simulink model "ASM_Traffic_V2X_Complete_Model_2"  (R2019a)
settings: Solver=ode1  StartTime=SIM.tstart.v  StopTime=Inf  FixedStep=SIM.StepSize.v  RelTol=1e-3
PostLoadFcn:
  | if any(exist('dsrtsu_mdlpostloadfcn', 'file') ~= 0), dsrtsu_mdlpostloadfcn('Execute', bdroot); end
  | try, asm_mdl_postloadfcn(bdroot, 'UpdateModel', 2200); catch, disp(lasterr); end,
undefined symbols (not defined in the file): _SensorPnts_1, _SensorPnts_13, _SensorPnts_17, _SensorPnts_21, _SensorPnts_25, _SensorPnts_29, _SensorPnts_33, _SensorPnts_37, _SensorPnts_41, _SensorPnts_45, _SensorPnts_49, _SensorPnts_5, _SensorPnts_53, _SensorPnts_57, _SensorPnts_9, _to_, CPT, G5A, ITS, MDL, rad, s_to_rpm, SIM
libraries: simulink x169, ASM_VehicleDynamics_lib x126, ASM_Traffic_lib x83, ASM_Utils_lib x49, mdbs x45, ASM_Environment_lib x17, dspindex x12, dsaV2xLibraryAux x10, dsmpblib x6, dsaV2xAsn1Library x4, dsaV2xLibrary x4, ASM_BrakeHydraulics_lib x4
(part 22 of 36)

== system ASM_Traffic_V2X_Complete_Model_2/MDLUserInterface/Environment/MDL_PAR/Fellow_VehicleLights/Fellow13_VehicleLights ==
  Bus Creator1 : BusCreator  Inputs=3
  SW_BrakeLight[0Off|1On] : Constant  Value=0
  SW_ManualControl_Lights[1Scheduler|2Manual] : Constant
  SW_TurnLights[0Off|1Left|2Right|3Both] : Constant  Value=0
  Out1 : Outport
  wires:
  SW_ManualControl_Lights[1Scheduler|2Manual]/1 -> Bus Creator1/1  "SW_ManualControl_Lights[1Scheduler|2Manual]"
  SW_TurnLights[0Off|1Left|2Right|3Both]/1 -> Bus Creator1/3  "SW_TurnLights[0Off|1Left|2Right|3Both]"
  SW_BrakeLight[0Off|1On]/1 -> Bus Creator1/2  "SW_BrakeLight[0Off|1On]"
  Bus Creator1/1 -> Out1/1

== system ASM_Traffic_V2X_Complete_Model_2/MDLUserInterface/Environment/MDL_PAR/Fellow_VehicleLights/Fellow14_VehicleLights ==
  Bus Creator1 : BusCreator  Inputs=3
  SW_BrakeLight[0Off|1On] : Constant  Value=0
  SW_ManualControl_Lights[1Scheduler|2Manual] : Constant
  SW_TurnLights[0Off|1Left|2Right|3Both] : Constant  Value=0
  Out1 : Outport
  wires:
  Bus Creator1/1 -> Out1/1
  SW_BrakeLight[0Off|1On]/1 -> Bus Creator1/2  "SW_BrakeLight[0Off|1On]"
  SW_TurnLights[0Off|1Left|2Right|3Both]/1 -> Bus Creator1/3  "SW_TurnLights[0Off|1Left|2Right|3Both]"
  SW_ManualControl_Lights[1Scheduler|2Manual]/1 -> Bus Creator1/1  "SW_ManualControl_Lights[1Scheduler|2Manual]"

== system ASM_Traffic_V2X_Complete_Model_2/MDLUserInterface/Environment/MDL_PAR/Fellow_VehicleLights/Fellow15_VehicleLights ==
  Bus Creator1 : BusCreator  Inputs=3
  SW_BrakeLight[0Off|1On] : Constant  Value=0
  SW_ManualControl_Lights[1Scheduler|2Manual] : Constant
  SW_TurnLights[0Off|1Left|2Right|3Both] : Constant  Value=0
  Out1 : Outport
  wires:
  SW_ManualControl_Lights[1Scheduler|2Manual]/1 -> Bus Creator1/1  "SW_ManualControl_Lights[1Scheduler|2Manual]"
  SW_TurnLights[0Off|1Left|2Right|3Both]/1 -> Bus Creator1/3  "SW_TurnLights[0Off|1Left|2Right|3Both]"
  SW_BrakeLight[0Off|1On]/1 -> Bus Creator1/2  "SW_BrakeLight[0Off|1On]"
  Bus Creator1/1 -> Out1/1

== system ASM_Traffic_V2X_Complete_Model_2/MDLUserInterface/Environment/MDL_PAR/Fellow_VehicleLights/Fellow1_VehicleLights ==
  Bus Creator1 : BusCreator  Inputs=3
  SW_BrakeLight[0Off|1On] : Constant  Value=0
  SW_ManualControl_Lights[1Scheduler|2Manual] : Constant
  SW_TurnLights[0Off|1Left|2Right|3Both] : Constant  Value=0
  Out1 : Outport
  wires:
  SW_ManualControl_Lights[1Scheduler|2Manual]/1 -> Bus Creator1/1  "SW_ManualControl_Lights[1Scheduler|2Manual]"
  SW_TurnLights[0Off|1Left|2Right|3Both]/1 -> Bus Creator1/3  "SW_TurnLights[0Off|1Left|2Right|3Both]"
  SW_BrakeLight[0Off|1On]/1 -> Bus Creator1/2  "SW_BrakeLight[0Off|1On]"
  Bus Creator1/1 -> Out1/1

== system ASM_Traffic_V2X_Complete_Model_2/MDLUserInterface/Environment/MDL_PAR/Fellow_VehicleLights/Fellow2_VehicleLights ==
  Bus Creator1 : BusCreator  Inputs=3
  SW_BrakeLight[0Off|1On] : Constant  Value=0
  SW_ManualControl_Lights[1Scheduler|2Manual] : Constant
  SW_TurnLights[0Off|1Left|2Right|3Both] : Constant  Value=0
  Out1 : Outport
  wires:
  Bus Creator1/1 -> Out1/1
  SW_BrakeLight[0Off|1On]/1 -> Bus Creator1/2  "SW_BrakeLight[0Off|1On]"
  SW_TurnLights[0Off|1Left|2Right|3Both]/1 -> Bus Creator1/3  "SW_TurnLights[0Off|1Left|2Right|3Both]"
  SW_ManualControl_Lights[1Scheduler|2Manual]/1 -> Bus Creator1/1  "SW_ManualControl_Lights[1Scheduler|2Manual]"

== system ASM_Traffic_V2X_Complete_Model_2/MDLUserInterface/Environment/MDL_PAR/Fellow_VehicleLights/Fellow3_VehicleLights ==
  Bus Creator1 : BusCreator  Inputs=3
  SW_BrakeLight[0Off|1On] : Constant  Value=0
  SW_ManualControl_Lights[1Scheduler|2Manual] : Constant
  SW_TurnLights[0Off|1Left|2Right|3Both] : Constant  Value=0
  Out1 : Outport
  wires:
  SW_ManualControl_Lights[1Scheduler|2Manual]/1 -> Bus Creator1/1  "SW_ManualControl_Lights[1Scheduler|2Manual]"
  SW_TurnLights[0Off|1Left|2Right|3Both]/1 -> Bus Creator1/3  "SW_TurnLights[0Off|1Left|2Right|3Both]"
  SW_BrakeLight[0Off|1On]/1 -> Bus Creator1/2  "SW_BrakeLight[0Off|1On]"
  Bus Creator1/1 -> Out1/1

== system ASM_Traffic_V2X_Complete_Model_2/MDLUserInterface/Environment/MDL_PAR/Fellow_VehicleLights/Fellow4_VehicleLights ==
  Bus Creator1 : BusCreator  Inputs=3
  SW_BrakeLight[0Off|1On] : Constant  Value=0
  SW_ManualControl_Lights[1Scheduler|2Manual] : Constant
  SW_TurnLights[0Off|1Left|2Right|3Both] : Constant  Value=0
  Out1 : Outport
  wires:
  Bus Creator1/1 -> Out1/1
  SW_BrakeLight[0Off|1On]/1 -> Bus Creator1/2  "SW_BrakeLight[0Off|1On]"
  SW_TurnLights[0Off|1Left|2Right|3Both]/1 -> Bus Creator1/3  "SW_TurnLights[0Off|1Left|2Right|3Both]"
  SW_ManualControl_Lights[1Scheduler|2Manual]/1 -> Bus Creator1/1  "SW_ManualControl_Lights[1Scheduler|2Manual]"

== system ASM_Traffic_V2X_Complete_Model_2/MDLUserInterface/Environment/MDL_PAR/Fellow_VehicleLights/Fellow5_VehicleLights ==
  Bus Creator1 : BusCreator  Inputs=3
  SW_BrakeLight[0Off|1On] : Constant  Value=0
  SW_ManualControl_Lights[1Scheduler|2Manual] : Constant
  SW_TurnLights[0Off|1Left|2Right|3Both] : Constant  Value=0
  Out1 : Outport
  wires:
  SW_ManualControl_Lights[1Scheduler|2Manual]/1 -> Bus Creator1/1  "SW_ManualControl_Lights[1Scheduler|2Manual]"
  SW_TurnLights[0Off|1Left|2Right|3Both]/1 -> Bus Creator1/3  "SW_TurnLights[0Off|1Left|2Right|3Both]"
  SW_BrakeLight[0Off|1On]/1 -> Bus Creator1/2  "SW_BrakeLight[0Off|1On]"
  Bus Creator1/1 -> Out1/1

== system ASM_Traffic_V2X_Complete_Model_2/MDLUserInterface/Environment/MDL_PAR/Fellow_VehicleLights/Fellow6_VehicleLights ==
  Bus Creator1 : BusCreator  Inputs=3
  SW_BrakeLight[0Off|1On] : Constant  Value=0
  SW_ManualControl_Lights[1Scheduler|2Manual] : Constant
  SW_TurnLights[0Off|1Left|2Right|3Both] : Constant  Value=0
  Out1 : Outport
  wires:
  Bus Creator1/1 -> Out1/1
  SW_BrakeLight[0Off|1On]/1 -> Bus Creator1/2  "SW_BrakeLight[0Off|1On]"
  SW_TurnLights[0Off|1Left|2Right|3Both]/1 -> Bus Creator1/3  "SW_TurnLights[0Off|1Left|2Right|3Both]"
  SW_ManualControl_Lights[1Scheduler|2Manual]/1 -> Bus Creator1/1  "SW_ManualControl_Lights[1Scheduler|2Manual]"

== system ASM_Traffic_V2X_Complete_Model_2/MDLUserInterface/Environment/MDL_PAR/Fellow_VehicleLights/Fellow7_VehicleLights ==
  Bus Creator1 : BusCreator  Inputs=3
  SW_BrakeLight[0Off|1On] : Constant  Value=0
  SW_ManualControl_Lights[1Scheduler|2Manual] : Constant
  SW_TurnLights[0Off|1Left|2Right|3Both] : Constant  Value=0
  Out1 : Outport
  wires:
  SW_ManualControl_Lights[1Scheduler|2Manual]/1 -> Bus Creator1/1  "SW_ManualControl_Lights[1Scheduler|2Manual]"
  SW_TurnLights[0Off|1Left|2Right|3Both]/1 -> Bus Creator1/3  "SW_TurnLights[0Off|1Left|2Right|3Both]"
  SW_BrakeLight[0Off|1On]/1 -> Bus Creator1/2  "SW_BrakeLight[0Off|1On]"
  Bus Creator1/1 -> Out1/1

== system ASM_Traffic_V2X_Complete_Model_2/MDLUserInterface/Environment/MDL_PAR/Fellow_VehicleLights/Fellow8_VehicleLights ==
  Bus Creator1 : BusCreator  Inputs=3
  SW_BrakeLight[0Off|1On] : Constant  Value=0
  SW_ManualControl_Lights[1Scheduler|2Manual] : Constant
  SW_TurnLights[0Off|1Left|2Right|3Both] : Constant  Value=0
  Out1 : Outport
  wires:
  Bus Creator1/1 -> Out1/1
  SW_BrakeLight[0Off|1On]/1 -> Bus Creator1/2  "SW_BrakeLight[0Off|1On]"
  SW_TurnLights[0Off|1Left|2Right|3Both]/1 -> Bus Creator1/3  "SW_TurnLights[0Off|1Left|2Right|3Both]"
  SW_ManualControl_Lights[1Scheduler|2Manual]/1 -> Bus Creator1/1  "SW_ManualControl_Lights[1Scheduler|2Manual]"

== system ASM_Traffic_V2X_Complete_Model_2/MDLUserInterface/Environment/MDL_PAR/Fellow_VehicleLights/Fellow9_VehicleLights ==
  Bus Creator1 : BusCreator  Inputs=3
  SW_BrakeLight[0Off|1On] : Constant  Value=0
  SW_ManualControl_Lights[1Scheduler|2Manual] : Constant
  SW_TurnLights[0Off|1Left|2Right|3Both] : Constant  Value=0
  Out1 : Outport
  wires:
  SW_ManualControl_Lights[1Scheduler|2Manual]/1 -> Bus Creator1/1  "SW_ManualControl_Lights[1Scheduler|2Manual]"
  SW_TurnLights[0Off|1Left|2Right|3Both]/1 -> Bus Creator1/3  "SW_TurnLights[0Off|1Left|2Right|3Both]"
  SW_BrakeLight[0Off|1On]/1 -> Bus Creator1/2  "SW_BrakeLight[0Off|1On]"
  Bus Creator1/1 -> Out1/1

== system ASM_Traffic_V2X_Complete_Model_2/MDLUserInterface/Environment/MDL_PAR/ManeuverControl/Enable_ManeuverStart ==
  Sw_StartManeuverAtSimStart[0|1] : Inport
  In : Inport  Port=2
  Data Type Conversion : DataTypeConversion
  Logical Operator : Logic  Operator=OR  AllPortsSameDT=off  OutDataTypeStr=boolean
  Product : Product  Inputs=3
  Step : Step  Time=0.005  SampleTime=0
  Step1 : Step  Time=0.02  Before=1  After=0  SampleTime=0
  Out : Outport
  wires:
  In/1 -> Logical Operator/1
  Data Type Conversion/1 -> Out/1
  Logical Operator/1 -> Data Type Conversion/1
  Step1/1 -> Product/3
  Product/1 -> Logical Operator/2
  Sw_StartManeuverAtSimStart[0|1]/1 -> Product/1
  Step/1 -> Product/2

== system ASM_Traffic_V2X_Complete_Model_2/MDLUserInterface/Environment/MDL_PAR/Objects_DataStreams/DataStream_1 ==
  Bus Creator1 : BusCreator  Inputs=4
  Ext_DataStream_1[] : Constant  Value=0
  Multiport Switch : MultiPortSwitch  DataPortOrder=Zero-based contiguous  Inputs=2  zeroidx=on
  Rounding Function : Rounding  Operator=round
  Saturation : Saturate  UpperLimit=2  LowerLimit=0
  Stim_DataStream_1[] : Constant
  Sw_DataStream_1[0Stim|1Ext] : Constant  Value=0
  DataStream_1[] : Outport
  wires:
  Sw_DataStream_1[0Stim|1Ext]/1 -> Rounding Function/1, Bus Creator1/1  "Sw_DataStream_1[0Stim|1Ext]"
  Ext_DataStream_1[]/1 -> Bus Creator1/3, Multiport Switch/3  "Ext_DataStream_1[]"
  Rounding Function/1 -> Saturation/1
  Saturation/1 -> Multiport Switch/1
  Multiport Switch/1 -> Bus Creator1/4  "DataStream_1[]"
  Stim_DataStream_1[]/1 -> Multiport Switch/2, Bus Creator1/2  "Stim_DataStream_1[]"
  Bus Creator1/1 -> DataStream_1[]/1

== system ASM_Traffic_V2X_Complete_Model_2/MDLUserInterface/Environment/MDL_PAR/Objects_DataStreams/DataStream_2 ==
  Bus Creator1 : BusCreator  Inputs=4
  Ext_DataStream_2[] : Constant  Value=0
  Multiport Switch : MultiPortSwitch  DataPortOrder=Zero-based contiguous  Inputs=2  zeroidx=on
  Rounding Function : Rounding  Operator=round
  Saturation : Saturate  UpperLimit=2  LowerLimit=0
  Stim_DataStream_2[] : Constant
  Sw_DataStream_2[0Stim|1Ext] : Constant  Value=0
  DataStream_2[] : Outport
  wires:
  Bus Creator1/1 -> DataStream_2[]/1
  Stim_DataStream_2[]/1 -> Bus Creator1/2, Multiport Switch/2  "Stim_DataStream_2[]"
  Multiport Switch/1 -> Bus Creator1/4  "DataStream_2[]"
  Saturation/1 -> Multiport Switch/1
  Rounding Function/1 -> Saturation/1
  Ext_DataStream_2[]/1 -> Multiport Switch/3, Bus Creator1/3  "Ext_DataStream_2[]"
  Sw_DataStream_2[0Stim|1Ext]/1 -> Bus Creator1/1, Rounding Function/1  "Sw_DataStream_2[0Stim|1Ext]"

== system ASM_Traffic_V2X_Complete_Model_2/MDLUserInterface/Environment/MDL_PAR/Objects_DataStreams/DataStream_3 ==
  Bus Creator1 : BusCreator  Inputs=4
  Ext_DataStream_3[] : Constant  Value=0
  Multiport Switch : MultiPortSwitch  DataPortOrder=Zero-based contiguous  Inputs=2  zeroidx=on
  Rounding Function : Rounding  Operator=round
  Saturation : Saturate  UpperLimit=2  LowerLimit=0
  Stim_DataStream_3[] : Constant
  Sw_DataStream_3[0Stim|1Ext] : Constant  Value=0
  DataStream_3[] : Outport
  wires:
  Sw_DataStream_3[0Stim|1Ext]/1 -> Rounding Function/1, Bus Creator1/1  "Sw_DataStream_3[0Stim|1Ext]"
  Ext_DataStream_3[]/1 -> Bus Creator1/3, Multiport Switch/3  "Ext_DataStream_3[]"
  Rounding Function/1 -> Saturation/1
  Saturation/1 -> Multiport Switch/1
  Multiport Switch/1 -> Bus Creator1/4  "DataStream_3[]"
  Stim_DataStream_3[]/1 -> Multiport Switch/2, Bus Creator1/2  "Stim_DataStream_3[]"
  Bus Creator1/1 -> DataStream_3[]/1

== system ASM_Traffic_V2X_Complete_Model_2/MDLUserInterface/Environment/MDL_PAR/Objects_DataStreams/DataStream_4 ==
  Bus Creator1 : BusCreator  Inputs=4
  Ext_DataStream_4[] : Constant  Value=0
  Multiport Switch : MultiPortSwitch  DataPortOrder=Zero-based contiguous  Inputs=2  zeroidx=on
  Rounding Function : Rounding  Operator=round
  Saturation : Saturate  UpperLimit=2  LowerLimit=0
  Stim_DataStream_4[] : Constant
  Sw_DataStream_4[0Stim|1Ext] : Constant  Value=0
  DataStream_4[] : Outport
  wires:
  Bus Creator1/1 -> DataStream_4[]/1
  Stim_DataStream_4[]/1 -> Bus Creator1/2, Multiport Switch/2  "Stim_DataStream_4[]"
  Multiport Switch/1 -> Bus Creator1/4  "DataStream_4[]"
  Saturation/1 -> Multiport Switch/1
  Rounding Function/1 -> Saturation/1
  Ext_DataStream_4[]/1 -> Multiport Switch/3, Bus Creator1/3  "Ext_DataStream_4[]"
  Sw_DataStream_4[0Stim|1Ext]/1 -> Bus Creator1/1, Rounding Function/1  "Sw_DataStream_4[0Stim|1Ext]"

== system ASM_Traffic_V2X_Complete_Model_2/MDLUserInterface/Environment/MDL_PAR/Objects_DataStreams/DataStream_5 ==
  Maneuver_Signals[] : Inport
  Bus Creator1 : BusCreator  Inputs=5
  Bus Selector2 : BusSelector  OutputSignals=UserSignals_Customized.Mnv_DataStream_5[]
  Ext_DataStream_5[] : Constant  Value=0
  Multiport Switch : MultiPortSwitch  DataPortOrder=Zero-based contiguous  zeroidx=on
  Rounding Function : Rounding  Operator=round
  Saturation : Saturate  UpperLimit=2  LowerLimit=0
  Stim_DataStream_5[] : Constant  Value=0
  Sw_DataStream_5[0Stim|1Ext|2Mnv] : Constant  Value=2
  DataStream_5[] : Outport
  wires:
  Sw_DataStream_5[0Stim|1Ext|2Mnv]/1 -> Rounding Function/1, Bus Creator1/1  "Sw_DataStream_5[0Stim|1Ext|2Mnv]"
  Maneuver_Signals[]/1 -> Bus Selector2/1
  Ext_DataStream_5[]/1 -> Multiport Switch/3, Bus Creator1/4  "Ext_DataStream_5[]"
  Bus Selector2/1 -> Multiport Switch/4, Bus Creator1/3  "<Mnv_DataStream_5[]>"
  Rounding Function/1 -> Saturation/1
  Saturation/1 -> Multiport Switch/1
  Multiport Switch/1 -> Bus Creator1/5  "DataStream_5[]"
  Stim_DataStream_5[]/1 -> Multiport Switch/2, Bus Creator1/2  "Stim_DataStream_5[]"
  Bus Creator1/1 -> DataStream_5[]/1

== system ASM_Traffic_V2X_Complete_Model_2/MDLUserInterface/Environment/MDL_PAR/Objects_DataStreams/DataStream_6 ==
  Maneuver_Signals[] : Inport
  Bus Creator1 : BusCreator  Inputs=5
  Bus Selector2 : BusSelector  OutputSignals=UserSignals_Customized.Mnv_DataStream_6[]
  Ext_DataStream_6[] : Constant  Value=0
  Multiport Switch : MultiPortSwitch  DataPortOrder=Zero-based contiguous  zeroidx=on
  Rounding Function : Rounding  Operator=round
  Saturation : Saturate  UpperLimit=2  LowerLimit=0
  Stim_DataStream_6[] : Constant  Value=0
  Sw_DataStream_6[0Stim|1Ext|2Mnv] : Constant  Value=2
  DataStream_6[] : Outport
  wires:
  Bus Creator1/1 -> DataStream_6[]/1
  Stim_DataStream_6[]/1 -> Bus Creator1/2, Multiport Switch/2  "Stim_DataStream_6[]"
  Multiport Switch/1 -> Bus Creator1/5  "DataStream_6[]"
  Saturation/1 -> Multiport Switch/1
  Rounding Function/1 -> Saturation/1
  Bus Selector2/1 -> Multiport Switch/4, Bus Creator1/3  "<Mnv_DataStream_6[]>"
  Ext_DataStream_6[]/1 -> Multiport Switch/3, Bus Creator1/4  "Ext_DataStream_6[]"
  Maneuver_Signals[]/1 -> Bus Selector2/1
  Sw_DataStream_6[0Stim|1Ext|2Mnv]/1 -> Bus Creator1/1, Rounding Function/1  "Sw_DataStream_6[0Stim|1Ext|2Mnv]"

== system ASM_Traffic_V2X_Complete_Model_2/MDLUserInterface/Environment/MDL_PAR/Objects_DataStreams/DataStream_7 ==
  Maneuver_Signals[] : Inport
  Bus Creator1 : BusCreator  Inputs=5
  Bus Selector2 : BusSelector  OutputSignals=UserSignals_Customized.Mnv_DataStream_7[]
  Ext_DataStream_7[] : Constant  Value=0
  Multiport Switch : MultiPortSwitch  DataPortOrder=Zero-based contiguous  zeroidx=on
  Rounding Function : Rounding  Operator=round
  Saturation : Saturate  UpperLimit=2  LowerLimit=0
  Stim_DataStream_7[] : Constant  Value=0
  Sw_DataStream_7[0Stim|1Ext|2Mnv] : Constant  Value=2
  DataStream_7[] : Outport
  wires:
  Sw_DataStream_7[0Stim|1Ext|2Mnv]/1 -> Rounding Function/1, Bus Creator1/1  "Sw_DataStream_7[0Stim|1Ext|2Mnv]"
  Maneuver_Signals[]/1 -> Bus Selector2/1
  Ext_DataStream_7[]/1 -> Multiport Switch/3, Bus Creator1/4  "Ext_DataStream_7[]"
  Bus Selector2/1 -> Multiport Switch/4, Bus Creator1/3  "<Mnv_DataStream_7[]>"
  Rounding Function/1 -> Saturation/1
  Saturation/1 -> Multiport Switch/1
  Multiport Switch/1 -> Bus Creator1/5  "DataStream_7[]"
  Stim_DataStream_7[]/1 -> Multiport Switch/2, Bus Creator1/2  "Stim_DataStream_7[]"
  Bus Creator1/1 -> DataStream_7[]/1

== system ASM_Traffic_V2X_Complete_Model_2/MDLUserInterface/Environment/MDL_PAR/Objects_DataStreams/DataStream_8 ==
  Maneuver_Signals[] : Inport
  Bus Creator1 : BusCreator  Inputs=5
  Bus Selector2 : BusSelector  OutputSignals=UserSignals_Customized.Mnv_DataStream_8[]
  Ext_DataStream_8[] : Constant  Value=0
  Multiport Switch : MultiPortSwitch  DataPortOrder=Zero-based contiguous  zeroidx=on
  Rounding Function : Rounding  Operator=round
  Saturation : Saturate  UpperLimit=2  LowerLimit=0
  Stim_DataStream_8[] : Constant  Value=0
  Sw_DataStream_8[0Stim|1Ext|2Mnv] : Constant  Value=2
  DataStream_8[] : Outport
  wires:
  Bus Creator1/1 -> DataStream_8[]/1
  Stim_DataStream_8[]/1 -> Bus Creator1/2, Multiport Switch/2  "Stim_DataStream_8[]"
  Multiport Switch/1 -> Bus Creator1/5  "DataStream_8[]"
  Saturation/1 -> Multiport Switch/1
  Rounding Function/1 -> Saturation/1
  Bus Selector2/1 -> Multiport Switch/4, Bus Creator1/3  "<Mnv_DataStream_8[]>"
  Ext_DataStream_8[]/1 -> Multiport Switch/3, Bus Creator1/4  "Ext_DataStream_8[]"
  Maneuver_Signals[]/1 -> Bus Selector2/1
  Sw_DataStream_8[0Stim|1Ext|2Mnv]/1 -> Bus Creator1/1, Rounding Function/1  "Sw_DataStream_8[0Stim|1Ext|2Mnv]"

== system ASM_Traffic_V2X_Complete_Model_2/MDLUserInterface/MotionDeskInterface/MOTION_DESK_INTERFACE/CalcLDWState/LeavingLane_L ==
  Action Port : ActionPort  ActionPortLabel=elseif((u1>0.01 & u1<=0.2))
  Constant : Constant  Value=2
  Out1 : Outport
  wires:
  Constant/1 -> Out1/1

== system ASM_Traffic_V2X_Complete_Model_2/MDLUserInterface/MotionDeskInterface/MOTION_DESK_INTERFACE/CalcLDWState/LeavingLane_R ==
  Action Port : ActionPort  ActionPortLabel=elseif((u1>0.01 & u1<=0.2))
  Constant : Constant  Value=2
  Out1 : Outport
  wires:
  Constant/1 -> Out1/1

== system ASM_Traffic_V2X_Complete_Model_2/MDLUserInterface/MotionDeskInterface/MOTION_DESK_INTERFACE/CalcLDWState/OK_L ==
  Action Port : ActionPort  ActionPortLabel=else
  Constant : Constant  Value=3
  Out1 : Outport
  wires:
  Constant/1 -> Out1/1

== system ASM_Traffic_V2X_Complete_Model_2/MDLUserInterface/MotionDeskInterface/MOTION_DESK_INTERFACE/CalcLDWState/OK_R ==
  Action Port : ActionPort  ActionPortLabel=else
  Constant : Constant  Value=3
  Out1 : Outport
  wires:
  Constant/1 -> Out1/1

== system ASM_Traffic_V2X_Complete_Model_2/MDLUserInterface/MotionDeskInterface/MOTION_DESK_INTERFACE/CalcLDWState/OutOfLane_L ==
  Action Port : ActionPort  ActionPortLabel=if(u1 <= 0.01)
  Constant : Constant
  Out1 : Outport
  wires:
  Constant/1 -> Out1/1

== system ASM_Traffic_V2X_Complete_Model_2/MDLUserInterface/MotionDeskInterface/MOTION_DESK_INTERFACE/CalcLDWState/OutOfLane_R ==
  Action Port : ActionPort  ActionPortLabel=if(u1 <= 0.01)
  Constant : Constant
  Out1 : Outport
  wires:
  Constant/1 -> Out1/1

== system ASM_Traffic_V2X_Complete_Model_2/MDLUserInterface/MotionDeskInterface/MOTION_DESK_INTERFACE/Coding/SwitchDelay ==
  Turnlight_L : Inport
  Turnlight_R : Inport  Port=2
  Add : Sum
  Compare To Constant : simulink/Logic and Bit Operations/Compare To Constant  relop=>  const=2  OutDataTypeStr=boolean
  Logical Operator1 : Logic  AllPortsSameDT=off  OutDataTypeStr=boolean
  Logical Operator2 : Logic  AllPortsSameDT=off  OutDataTypeStr=boolean
  Logical Operator4 : Logic  AllPortsSameDT=off  OutDataTypeStr=boolean
  Relational Operator3 : RelationalOperator  Operator=>  OutDataTypeStr=boolean  RndMeth=Nearest
  Switch : Switch  Criteria=u2 > Threshold
  Unit Delay{1..3,6} (4 alike) : UnitDelay  SampleTime=-1
  one : Constant  OutDataTypeStr=uint32
  zero : Constant  Value=0  OutDataTypeStr=uint32
  Turnlight_L_out : Outport
  Turnlight_R_out : Outport  Port=2
  wires:
  Unit Delay6/1 -> Logical Operator4/1
  Unit Delay3/1 -> Logical Operator2/1
  Unit Delay2/1 -> Relational Operator3/2
  Logical Operator1/1 -> Relational Operator3/1, Unit Delay2/1
  Relational Operator3/1 -> Switch/2
  zero/1 -> Switch/1
  Switch/1 -> Unit Delay1/1
  one/1 -> Add/1
  Unit Delay1/1 -> Add/2, Compare To Constant/1
  Add/1 -> Switch/3
  Compare To Constant/1 -> Logical Operator2/2, Logical Operator4/2
  Logical Operator2/1 -> Turnlight_L_out/1
  Logical Operator4/1 -> Turnlight_R_out/1
  Turnlight_L/1 -> Unit Delay3/1, Logical Operator1/1
  Turnlight_R/1 -> Unit Delay6/1, Logical Operator1/2

== system ASM_Traffic_V2X_Complete_Model_2/MDLUserInterface/MotionDeskInterface/MOTION_DESK_INTERFACE/Coding_Fellows/Coding1 ==
  In1 : Inport
  Bitwise Operator3 : simulink/Logic and Bit Operations/Bitwise Operator  logicop=OR  UseBitMask=off  NumInputPorts=3  BitMask=bin2dec('11011001')  BitMaskRealWorld=Stored Integer
  Data Type Conversion : DataTypeConversion  OutDataTypeStr=uint32
  Data Type Conversion1 : DataTypeConversion  OutDataTypeStr=uint32
  Demux : Demux  Outputs=3
  Gain : Gain  Gain=15  ParamDataTypeStr=uint32  OutDataTypeStr=uint32
  Gain1 : Gain  Gain=15  ParamDataTypeStr=uint32  OutDataTypeStr=uint32
  Gain2 : Gain  Gain=15  ParamDataTypeStr=uint32  OutDataTypeStr=uint32
  Shift Arithmetic : ArithShift  BitShiftNumber=4  BitShiftDirection=Left
  Shift Arithmetic1 : ArithShift  BitShiftNumber=8  BitShiftDirection=Left
  SwitchDelay : Subsystem
  Out1 : Outport
  wires:
  Data Type Conversion1/1 -> Out1/1
  Bitwise Operator3/1 -> Data Type Conversion1/1
  Demux/1 -> Gain/1
  Data Type Conversion/1 -> Demux/1
  Shift Arithmetic1/1 -> Bitwise Operator3/3
  Shift Arithmetic/1 -> Bitwise Operator3/2
  Gain2/1 -> Shift Arithmetic1/1
  Gain1/1 -> Shift Arithmetic/1
  Gain/1 -> Bitwise Operator3/1
  In1/1 -> Data Type Conversion/1
  Demux/2 -> SwitchDelay/1(Turnlight_L)
  Demux/3 -> SwitchDelay/2(Turnlight_R)
  SwitchDelay/1(Turnlight_L_out) -> Gain1/1
  SwitchDelay/2(Turnlight_R_out) -> Gain2/1

== system ASM_Traffic_V2X_Complete_Model_2/MDLUserInterface/MotionDeskInterface/MOTION_DESK_INTERFACE/Coding_Fellows/Coding10 ==
  In1 : Inport
  Bitwise Operator3 : simulink/Logic and Bit Operations/Bitwise Operator  logicop=OR  UseBitMask=off  NumInputPorts=3  BitMask=bin2dec('11011001')  BitMaskRealWorld=Stored Integer
  Data Type Conversion : DataTypeConversion  OutDataTypeStr=uint32
  Data Type Conversion1 : DataTypeConversion  OutDataTypeStr=uint32
  Demux : Demux  Outputs=3
  Gain : Gain  Gain=15  ParamDataTypeStr=uint32  OutDataTypeStr=uint32
  Gain1 : Gain  Gain=15  ParamDataTypeStr=uint32  OutDataTypeStr=uint32
  Gain2 : Gain  Gain=15  ParamDataTypeStr=uint32  OutDataTypeStr=uint32
  Shift Arithmetic : ArithShift  BitShiftNumber=4  BitShiftDirection=Left
  Shift Arithmetic1 : ArithShift  BitShiftNumber=8  BitShiftDirection=Left
  SwitchDelay : Subsystem
  Out1 : Outport
  wires:
  SwitchDelay/2(Turnlight_R_out) -> Gain2/1
  SwitchDelay/1(Turnlight_L_out) -> Gain1/1
  Demux/3 -> SwitchDelay/2(Turnlight_R)
  Demux/2 -> SwitchDelay/1(Turnlight_L)
  In1/1 -> Data Type Conversion/1
  Gain/1 -> Bitwise Operator3/1
  Gain1/1 -> Shift Arithmetic/1
  Gain2/1 -> Shift Arithmetic1/1
  Shift Arithmetic/1 -> Bitwise Operator3/2
  Shift Arithmetic1/1 -> Bitwise Operator3/3
  Data Type Conversion/1 -> Demux/1
  Demux/1 -> Gain/1
  Bitwise Operator3/1 -> Data Type Conversion1/1
  Data Type Conversion1/1 -> Out1/1

== system ASM_Traffic_V2X_Complete_Model_2/MDLUserInterface/MotionDeskInterface/MOTION_DESK_INTERFACE/Coding_Fellows/Coding11 ==
  In1 : Inport
  Bitwise Operator3 : simulink/Logic and Bit Operations/Bitwise Operator  logicop=OR  UseBitMask=off  NumInputPorts=3  BitMask=bin2dec('11011001')  BitMaskRealWorld=Stored Integer
  Data Type Conversion : DataTypeConversion  OutDataTypeStr=uint32
  Data Type Conversion1 : DataTypeConversion  OutDataTypeStr=uint32
  Demux : Demux  Outputs=3
  Gain : Gain  Gain=15  ParamDataTypeStr=uint32  OutDataTypeStr=uint32
  Gain1 : Gain  Gain=15  ParamDataTypeStr=uint32  OutDataTypeStr=uint32
  Gain2 : Gain  Gain=15  ParamDataTypeStr=uint32  OutDataTypeStr=uint32
  Shift Arithmetic : ArithShift  BitShiftNumber=4  BitShiftDirection=Left
  Shift Arithmetic1 : ArithShift  BitShiftNumber=8  BitShiftDirection=Left
  SwitchDelay : Subsystem
  Out1 : Outport
  wires:
  Data Type Conversion1/1 -> Out1/1
  Bitwise Operator3/1 -> Data Type Conversion1/1
  Demux/1 -> Gain/1
  Data Type Conversion/1 -> Demux/1
  Shift Arithmetic1/1 -> Bitwise Operator3/3
  Shift Arithmetic/1 -> Bitwise Operator3/2
  Gain2/1 -> Shift Arithmetic1/1
  Gain1/1 -> Shift Arithmetic/1
  Gain/1 -> Bitwise Operator3/1
  In1/1 -> Data Type Conversion/1
  Demux/2 -> SwitchDelay/1(Turnlight_L)
  Demux/3 -> SwitchDelay/2(Turnlight_R)
  SwitchDelay/1(Turnlight_L_out) -> Gain1/1
  SwitchDelay/2(Turnlight_R_out) -> Gain2/1

== system ASM_Traffic_V2X_Complete_Model_2/MDLUserInterface/MotionDeskInterface/MOTION_DESK_INTERFACE/Coding_Fellows/Coding12 ==
  In1 : Inport
  Bitwise Operator3 : simulink/Logic and Bit Operations/Bitwise Operator  logicop=OR  UseBitMask=off  NumInputPorts=3  BitMask=bin2dec('11011001')  BitMaskRealWorld=Stored Integer
  Data Type Conversion : DataTypeConversion  OutDataTypeStr=uint32
  Data Type Conversion1 : DataTypeConversion  OutDataTypeStr=uint32
  Demux : Demux  Outputs=3
  Gain : Gain  Gain=15  ParamDataTypeStr=uint32  OutDataTypeStr=uint32
  Gain1 : Gain  Gain=15  ParamDataTypeStr=uint32  OutDataTypeStr=uint32
  Gain2 : Gain  Gain=15  ParamDataTypeStr=uint32  OutDataTypeStr=uint32
  Shift Arithmetic : ArithShift  BitShiftNumber=4  BitShiftDirection=Left
  Shift Arithmetic1 : ArithShift  BitShiftNumber=8  BitShiftDirection=Left
  SwitchDelay : Subsystem
  Out1 : Outport
  wires:
  SwitchDelay/2(Turnlight_R_out) -> Gain2/1
  SwitchDelay/1(Turnlight_L_out) -> Gain1/1
  Demux/3 -> SwitchDelay/2(Turnlight_R)
  Demux/2 -> SwitchDelay/1(Turnlight_L)
  In1/1 -> Data Type Conversion/1
  Gain/1 -> Bitwise Operator3/1
  Gain1/1 -> Shift Arithmetic/1
  Gain2/1 -> Shift Arithmetic1/1
  Shift Arithmetic/1 -> Bitwise Operator3/2
  Shift Arithmetic1/1 -> Bitwise Operator3/3
  Data Type Conversion/1 -> Demux/1
  Demux/1 -> Gain/1
  Bitwise Operator3/1 -> Data Type Conversion1/1
  Data Type Conversion1/1 -> Out1/1

== system ASM_Traffic_V2X_Complete_Model_2/MDLUserInterface/MotionDeskInterface/MOTION_DESK_INTERFACE/Coding_Fellows/Coding13 ==
  In1 : Inport
  Bitwise Operator3 : simulink/Logic and Bit Operations/Bitwise Operator  logicop=OR  UseBitMask=off  NumInputPorts=3  BitMask=bin2dec('11011001')  BitMaskRealWorld=Stored Integer
  Data Type Conversion : DataTypeConversion  OutDataTypeStr=uint32
  Data Type Conversion1 : DataTypeConversion  OutDataTypeStr=uint32
  Demux : Demux  Outputs=3
  Gain : Gain  Gain=15  ParamDataTypeStr=uint32  OutDataTypeStr=uint32
  Gain1 : Gain  Gain=15  ParamDataTypeStr=uint32  OutDataTypeStr=uint32
  Gain2 : Gain  Gain=15  ParamDataTypeStr=uint32  OutDataTypeStr=uint32
  Shift Arithmetic : ArithShift  BitShiftNumber=4  BitShiftDirection=Left
  Shift Arithmetic1 : ArithShift  BitShiftNumber=8  BitShiftDirection=Left
  SwitchDelay : Subsystem
  Out1 : Outport
  wires:
  Data Type Conversion1/1 -> Out1/1
  Bitwise Operator3/1 -> Data Type Conversion1/1
  Demux/1 -> Gain/1
  Data Type Conversion/1 -> Demux/1
  Shift Arithmetic1/1 -> Bitwise Operator3/3
  Shift Arithmetic/1 -> Bitwise Operator3/2
  Gain2/1 -> Shift Arithmetic1/1
  Gain1/1 -> Shift Arithmetic/1
  Gain/1 -> Bitwise Operator3/1
  In1/1 -> Data Type Conversion/1
  Demux/2 -> SwitchDelay/1(Turnlight_L)
  Demux/3 -> SwitchDelay/2(Turnlight_R)
  SwitchDelay/1(Turnlight_L_out) -> Gain1/1
  SwitchDelay/2(Turnlight_R_out) -> Gain2/1

== system ASM_Traffic_V2X_Complete_Model_2/MDLUserInterface/MotionDeskInterface/MOTION_DESK_INTERFACE/Coding_Fellows/Coding14 ==
  In1 : Inport
  Bitwise Operator3 : simulink/Logic and Bit Operations/Bitwise Operator  logicop=OR  UseBitMask=off  NumInputPorts=3  BitMask=bin2dec('11011001')  BitMaskRealWorld=Stored Integer
  Data Type Conversion : DataTypeConversion  OutDataTypeStr=uint32
  Data Type Conversion1 : DataTypeConversion  OutDataTypeStr=uint32
  Demux : Demux  Outputs=3
  Gain : Gain  Gain=15  ParamDataTypeStr=uint32  OutDataTypeStr=uint32
  Gain1 : Gain  Gain=15  ParamDataTypeStr=uint32  OutDataTypeStr=uint32
  Gain2 : Gain  Gain=15  ParamDataTypeStr=uint32  OutDataTypeStr=uint32
  Shift Arithmetic : ArithShift  BitShiftNumber=4  BitShiftDirection=Left
  Shift Arithmetic1 : ArithShift  BitShiftNumber=8  BitShiftDirection=Left
  SwitchDelay : Subsystem
  Out1 : Outport
  wires:
  SwitchDelay/2(Turnlight_R_out) -> Gain2/1
  SwitchDelay/1(Turnlight_L_out) -> Gain1/1
  Demux/3 -> SwitchDelay/2(Turnlight_R)
  Demux/2 -> SwitchDelay/1(Turnlight_L)
  In1/1 -> Data Type Conversion/1
  Gain/1 -> Bitwise Operator3/1
  Gain1/1 -> Shift Arithmetic/1
  Gain2/1 -> Shift Arithmetic1/1
  Shift Arithmetic/1 -> Bitwise Operator3/2
  Shift Arithmetic1/1 -> Bitwise Operator3/3
  Data Type Conversion/1 -> Demux/1
  Demux/1 -> Gain/1
  Bitwise Operator3/1 -> Data Type Conversion1/1
  Data Type Conversion1/1 -> Out1/1

== system ASM_Traffic_V2X_Complete_Model_2/MDLUserInterface/MotionDeskInterface/MOTION_DESK_INTERFACE/Coding_Fellows/Coding15 ==
  In1 : Inport
  Bitwise Operator3 : simulink/Logic and Bit Operations/Bitwise Operator  logicop=OR  UseBitMask=off  NumInputPorts=3  BitMask=bin2dec('11011001')  BitMaskRealWorld=Stored Integer
  Data Type Conversion : DataTypeConversion  OutDataTypeStr=uint32
  Data Type Conversion1 : DataTypeConversion  OutDataTypeStr=uint32
  Demux : Demux  Outputs=3
  Gain : Gain  Gain=15  ParamDataTypeStr=uint32  OutDataTypeStr=uint32
  Gain1 : Gain  Gain=15  ParamDataTypeStr=uint32  OutDataTypeStr=uint32
  Gain2 : Gain  Gain=15  ParamDataTypeStr=uint32  OutDataTypeStr=uint32
  Shift Arithmetic : ArithShift  BitShiftNumber=4  BitShiftDirection=Left
  Shift Arithmetic1 : ArithShift  BitShiftNumber=8  BitShiftDirection=Left
  SwitchDelay : Subsystem
  Out1 : Outport
  wires:
  Data Type Conversion1/1 -> Out1/1
  Bitwise Operator3/1 -> Data Type Conversion1/1
  Demux/1 -> Gain/1
  Data Type Conversion/1 -> Demux/1
  Shift Arithmetic1/1 -> Bitwise Operator3/3
  Shift Arithmetic/1 -> Bitwise Operator3/2
  Gain2/1 -> Shift Arithmetic1/1
  Gain1/1 -> Shift Arithmetic/1
  Gain/1 -> Bitwise Operator3/1
  In1/1 -> Data Type Conversion/1
  Demux/2 -> SwitchDelay/1(Turnlight_L)
  Demux/3 -> SwitchDelay/2(Turnlight_R)
  SwitchDelay/1(Turnlight_L_out) -> Gain1/1
  SwitchDelay/2(Turnlight_R_out) -> Gain2/1

== system ASM_Traffic_V2X_Complete_Model_2/MDLUserInterface/MotionDeskInterface/MOTION_DESK_INTERFACE/Coding_Fellows/Coding2 ==
  In1 : Inport
  Bitwise Operator3 : simulink/Logic and Bit Operations/Bitwise Operator  logicop=OR  UseBitMask=off  NumInputPorts=3  BitMask=bin2dec('11011001')  BitMaskRealWorld=Stored Integer
  Data Type Conversion : DataTypeConversion  OutDataTypeStr=uint32
  Data Type Conversion1 : DataTypeConversion  OutDataTypeStr=uint32
  Demux : Demux  Outputs=3
  Gain : Gain  Gain=15  ParamDataTypeStr=uint32  OutDataTypeStr=uint32
  Gain1 : Gain  Gain=15  ParamDataTypeStr=uint32  OutDataTypeStr=uint32
  Gain2 : Gain  Gain=15  ParamDataTypeStr=uint32  OutDataTypeStr=uint32
  Shift Arithmetic : ArithShift  BitShiftNumber=4  BitShiftDirection=Left
  Shift Arithmetic1 : ArithShift  BitShiftNumber=8  BitShiftDirection=Left
  SwitchDelay : Subsystem
  Out1 : Outport
  wires:
  SwitchDelay/2(Turnlight_R_out) -> Gain2/1
  SwitchDelay/1(Turnlight_L_out) -> Gain1/1
  Demux/3 -> SwitchDelay/2(Turnlight_R)
  Demux/2 -> SwitchDelay/1(Turnlight_L)
  In1/1 -> Data Type Conversion/1
  Gain/1 -> Bitwise Operator3/1
  Gain1/1 -> Shift Arithmetic/1
  Gain2/1 -> Shift Arithmetic1/1
  Shift Arithmetic/1 -> Bitwise Operator3/2
  Shift Arithmetic1/1 -> Bitwise Operator3/3
  Data Type Conversion/1 -> Demux/1
  Demux/1 -> Gain/1
  Bitwise Operator3/1 -> Data Type Conversion1/1
  Data Type Conversion1/1 -> Out1/1

== system ASM_Traffic_V2X_Complete_Model_2/MDLUserInterface/MotionDeskInterface/MOTION_DESK_INTERFACE/Coding_Fellows/Coding3 ==
  In1 : Inport
  Bitwise Operator3 : simulink/Logic and Bit Operations/Bitwise Operator  logicop=OR  UseBitMask=off  NumInputPorts=3  BitMask=bin2dec('11011001')  BitMaskRealWorld=Stored Integer
  Data Type Conversion : DataTypeConversion  OutDataTypeStr=uint32
  Data Type Conversion1 : DataTypeConversion  OutDataTypeStr=uint32
  Demux : Demux  Outputs=3
  Gain : Gain  Gain=15  ParamDataTypeStr=uint32  OutDataTypeStr=uint32
  Gain1 : Gain  Gain=15  ParamDataTypeStr=uint32  OutDataTypeStr=uint32
  Gain2 : Gain  Gain=15  ParamDataTypeStr=uint32  OutDataTypeStr=uint32
  Shift Arithmetic : ArithShift  BitShiftNumber=4  BitShiftDirection=Left
  Shift Arithmetic1 : ArithShift  BitShiftNumber=8  BitShiftDirection=Left
  SwitchDelay : Subsystem
  Out1 : Outport
  wires:
  Data Type Conversion1/1 -> Out1/1
  Bitwise Operator3/1 -> Data Type Conversion1/1
  Demux/1 -> Gain/1
  Data Type Conversion/1 -> Demux/1
  Shift Arithmetic1/1 -> Bitwise Operator3/3
  Shift Arithmetic/1 -> Bitwise Operator3/2
  Gain2/1 -> Shift Arithmetic1/1
  Gain1/1 -> Shift Arithmetic/1
  Gain/1 -> Bitwise Operator3/1
  In1/1 -> Data Type Conversion/1
  Demux/2 -> SwitchDelay/1(Turnlight_L)
  Demux/3 -> SwitchDelay/2(Turnlight_R)
  SwitchDelay/1(Turnlight_L_out) -> Gain1/1
  SwitchDelay/2(Turnlight_R_out) -> Gain2/1

== system ASM_Traffic_V2X_Complete_Model_2/MDLUserInterface/MotionDeskInterface/MOTION_DESK_INTERFACE/Coding_Fellows/Coding4 ==
  In1 : Inport
  Bitwise Operator3 : simulink/Logic and Bit Operations/Bitwise Operator  logicop=OR  UseBitMask=off  NumInputPorts=3  BitMask=bin2dec('11011001')  BitMaskRealWorld=Stored Integer
  Data Type Conversion : DataTypeConversion  OutDataTypeStr=uint32
  Data Type Conversion1 : DataTypeConversion  OutDataTypeStr=uint32
  Demux : Demux  Outputs=3
  Gain : Gain  Gain=15  ParamDataTypeStr=uint32  OutDataTypeStr=uint32
  Gain1 : Gain  Gain=15  ParamDataTypeStr=uint32  OutDataTypeStr=uint32
  Gain2 : Gain  Gain=15  ParamDataTypeStr=uint32  OutDataTypeStr=uint32
  Shift Arithmetic : ArithShift  BitShiftNumber=4  BitShiftDirection=Left
  Shift Arithmetic1 : ArithShift  BitShiftNumber=8  BitShiftDirection=Left
  SwitchDelay : Subsystem
  Out1 : Outport
  wires:
  SwitchDelay/2(Turnlight_R_out) -> Gain2/1
  SwitchDelay/1(Turnlight_L_out) -> Gain1/1
  Demux/3 -> SwitchDelay/2(Turnlight_R)
  Demux/2 -> SwitchDelay/1(Turnlight_L)
  In1/1 -> Data Type Conversion/1
  Gain/1 -> Bitwise Operator3/1
  Gain1/1 -> Shift Arithmetic/1
  Gain2/1 -> Shift Arithmetic1/1
  Shift Arithmetic/1 -> Bitwise Operator3/2
  Shift Arithmetic1/1 -> Bitwise Operator3/3
  Data Type Conversion/1 -> Demux/1
  Demux/1 -> Gain/1
  Bitwise Operator3/1 -> Data Type Conversion1/1
  Data Type Conversion1/1 -> Out1/1

== system ASM_Traffic_V2X_Complete_Model_2/MDLUserInterface/MotionDeskInterface/MOTION_DESK_INTERFACE/Coding_Fellows/Coding5 ==
  In1 : Inport
  Bitwise Operator3 : simulink/Logic and Bit Operations/Bitwise Operator  logicop=OR  UseBitMask=off  NumInputPorts=3  BitMask=bin2dec('11011001')  BitMaskRealWorld=Stored Integer
  Data Type Conversion : DataTypeConversion  OutDataTypeStr=uint32
  Data Type Conversion1 : DataTypeConversion  OutDataTypeStr=uint32
  Demux : Demux  Outputs=3
  Gain : Gain  Gain=15  ParamDataTypeStr=uint32  OutDataTypeStr=uint32
  Gain1 : Gain  Gain=15  ParamDataTypeStr=uint32  OutDataTypeStr=uint32
  Gain2 : Gain  Gain=15  ParamDataTypeStr=uint32  OutDataTypeStr=uint32
  Shift Arithmetic : ArithShift  BitShiftNumber=4  BitShiftDirection=Left
  Shift Arithmetic1 : ArithShift  BitShiftNumber=8  BitShiftDirection=Left
  SwitchDelay : Subsystem
  Out1 : Outport
  wires:
  Data Type Conversion1/1 -> Out1/1
  Bitwise Operator3/1 -> Data Type Conversion1/1
  Demux/1 -> Gain/1
  Data Type Conversion/1 -> Demux/1
  Shift Arithmetic1/1 -> Bitwise Operator3/3
  Shift Arithmetic/1 -> Bitwise Operator3/2
  Gain2/1 -> Shift Arithmetic1/1
  Gain1/1 -> Shift Arithmetic/1
  Gain/1 -> Bitwise Operator3/1
  In1/1 -> Data Type Conversion/1
  Demux/2 -> SwitchDelay/1(Turnlight_L)
  Demux/3 -> SwitchDelay/2(Turnlight_R)
  SwitchDelay/1(Turnlight_L_out) -> Gain1/1
  SwitchDelay/2(Turnlight_R_out) -> Gain2/1

== system ASM_Traffic_V2X_Complete_Model_2/MDLUserInterface/MotionDeskInterface/MOTION_DESK_INTERFACE/Coding_Fellows/Coding6 ==
  In1 : Inport
  Bitwise Operator3 : simulink/Logic and Bit Operations/Bitwise Operator  logicop=OR  UseBitMask=off  NumInputPorts=3  BitMask=bin2dec('11011001')  BitMaskRealWorld=Stored Integer
  Data Type Conversion : DataTypeConversion  OutDataTypeStr=uint32
  Data Type Conversion1 : DataTypeConversion  OutDataTypeStr=uint32
  Demux : Demux  Outputs=3
  Gain : Gain  Gain=15  ParamDataTypeStr=uint32  OutDataTypeStr=uint32
  Gain1 : Gain  Gain=15  ParamDataTypeStr=uint32  OutDataTypeStr=uint32
  Gain2 : Gain  Gain=15  ParamDataTypeStr=uint32  OutDataTypeStr=uint32
  Shift Arithmetic : ArithShift  BitShiftNumber=4  BitShiftDirection=Left
  Shift Arithmetic1 : ArithShift  BitShiftNumber=8  BitShiftDirection=Left
  SwitchDelay : Subsystem
  Out1 : Outport
  wires:
  SwitchDelay/2(Turnlight_R_out) -> Gain2/1
  SwitchDelay/1(Turnlight_L_out) -> Gain1/1
  Demux/3 -> SwitchDelay/2(Turnlight_R)
  Demux/2 -> SwitchDelay/1(Turnlight_L)
  In1/1 -> Data Type Conversion/1
  Gain/1 -> Bitwise Operator3/1
  Gain1/1 -> Shift Arithmetic/1
  Gain2/1 -> Shift Arithmetic1/1
  Shift Arithmetic/1 -> Bitwise Operator3/2
  Shift Arithmetic1/1 -> Bitwise Operator3/3
  Data Type Conversion/1 -> Demux/1
  Demux/1 -> Gain/1
  Bitwise Operator3/1 -> Data Type Conversion1/1
  Data Type Conversion1/1 -> Out1/1

== system ASM_Traffic_V2X_Complete_Model_2/MDLUserInterface/MotionDeskInterface/MOTION_DESK_INTERFACE/Coding_Fellows/Coding7 ==
  In1 : Inport
  Bitwise Operator3 : simulink/Logic and Bit Operations/Bitwise Operator  logicop=OR  UseBitMask=off  NumInputPorts=3  BitMask=bin2dec('11011001')  BitMaskRealWorld=Stored Integer
  Data Type Conversion : DataTypeConversion  OutDataTypeStr=uint32
  Data Type Conversion1 : DataTypeConversion  OutDataTypeStr=uint32
  Demux : Demux  Outputs=3
  Gain : Gain  Gain=15  ParamDataTypeStr=uint32  OutDataTypeStr=uint32
  Gain1 : Gain  Gain=15  ParamDataTypeStr=uint32  OutDataTypeStr=uint32
  Gain2 : Gain  Gain=15  ParamDataTypeStr=uint32  OutDataTypeStr=uint32
  Shift Arithmetic : ArithShift  BitShiftNumber=4  BitShiftDirection=Left
  Shift Arithmetic1 : ArithShift  BitShiftNumber=8  BitShiftDirection=Left
  SwitchDelay : Subsystem
  Out1 : Outport
  wires:
  Data Type Conversion1/1 -> Out1/1
  Bitwise Operator3/1 -> Data Type Conversion1/1
  Demux/1 -> Gain/1
  Data Type Conversion/1 -> Demux/1
  Shift Arithmetic1/1 -> Bitwise Operator3/3
  Shift Arithmetic/1 -> Bitwise Operator3/2
  Gain2/1 -> Shift Arithmetic1/1
  Gain1/1 -> Shift Arithmetic/1
  Gain/1 -> Bitwise Operator3/1
  In1/1 -> Data Type Conversion/1
  Demux/2 -> SwitchDelay/1(Turnlight_L)
  Demux/3 -> SwitchDelay/2(Turnlight_R)
  SwitchDelay/1(Turnlight_L_out) -> Gain1/1
  SwitchDelay/2(Turnlight_R_out) -> Gain2/1

== system ASM_Traffic_V2X_Complete_Model_2/MDLUserInterface/MotionDeskInterface/MOTION_DESK_INTERFACE/Coding_Fellows/Coding8 ==
  In1 : Inport
  Bitwise Operator3 : simulink/Logic and Bit Operations/Bitwise Operator  logicop=OR  UseBitMask=off  NumInputPorts=3  BitMask=bin2dec('11011001')  BitMaskRealWorld=Stored Integer
  Data Type Conversion : DataTypeConversion  OutDataTypeStr=uint32
  Data Type Conversion1 : DataTypeConversion  OutDataTypeStr=uint32
  Demux : Demux  Outputs=3
  Gain : Gain  Gain=15  ParamDataTypeStr=uint32  OutDataTypeStr=uint32
  Gain1 : Gain  Gain=15  ParamDataTypeStr=uint32  OutDataTypeStr=uint32
  Gain2 : Gain  Gain=15  ParamDataTypeStr=uint32  OutDataTypeStr=uint32
  Shift Arithmetic : ArithShift  BitShiftNumber=4  BitShiftDirection=Left
  Shift Arithmetic1 : ArithShift  BitShiftNumber=8  BitShiftDirection=Left
  SwitchDelay : Subsystem
  Out1 : Outport
  wires:
  SwitchDelay/2(Turnlight_R_out) -> Gain2/1
  SwitchDelay/1(Turnlight_L_out) -> Gain1/1
  Demux/3 -> SwitchDelay/2(Turnlight_R)
  Demux/2 -> SwitchDelay/1(Turnlight_L)
  In1/1 -> Data Type Conversion/1
  Gain/1 -> Bitwise Operator3/1
  Gain1/1 -> Shift Arithmetic/1
  Gain2/1 -> Shift Arithmetic1/1
  Shift Arithmetic/1 -> Bitwise Operator3/2
  Shift Arithmetic1/1 -> Bitwise Operator3/3
  Data Type Conversion/1 -> Demux/1
  Demux/1 -> Gain/1
  Bitwise Operator3/1 -> Data Type Conversion1/1
  Data Type Conversion1/1 -> Out1/1

== system ASM_Traffic_V2X_Complete_Model_2/MDLUserInterface/MotionDeskInterface/MOTION_DESK_INTERFACE/Coding_Fellows/Coding9 ==
  In1 : Inport
  Bitwise Operator3 : simulink/Logic and Bit Operations/Bitwise Operator  logicop=OR  UseBitMask=off  NumInputPorts=3  BitMask=bin2dec('11011001')  BitMaskRealWorld=Stored Integer
  Data Type Conversion : DataTypeConversion  OutDataTypeStr=uint32
  Data Type Conversion1 : DataTypeConversion  OutDataTypeStr=uint32
  Demux : Demux  Outputs=3
  Gain : Gain  Gain=15  ParamDataTypeStr=uint32  OutDataTypeStr=uint32
  Gain1 : Gain  Gain=15  ParamDataTypeStr=uint32  OutDataTypeStr=uint32
  Gain2 : Gain  Gain=15  ParamDataTypeStr=uint32  OutDataTypeStr=uint32
  Shift Arithmetic : ArithShift  BitShiftNumber=4  BitShiftDirection=Left
  Shift Arithmetic1 : ArithShift  BitShiftNumber=8  BitShiftDirection=Left
  SwitchDelay : Subsystem
  Out1 : Outport
  wires:
  Data Type Conversion1/1 -> Out1/1
  Bitwise Operator3/1 -> Data Type Conversion1/1
  Demux/1 -> Gain/1
  Data Type Conversion/1 -> Demux/1
  Shift Arithmetic1/1 -> Bitwise Operator3/3
  Shift Arithmetic/1 -> Bitwise Operator3/2
  Gain2/1 -> Shift Arithmetic1/1
  Gain1/1 -> Shift Arithmetic/1
  Gain/1 -> Bitwise Operator3/1
  In1/1 -> Data Type Conversion/1
  Demux/2 -> SwitchDelay/1(Turnlight_L)
  Demux/3 -> SwitchDelay/2(Turnlight_R)
  SwitchDelay/1(Turnlight_L_out) -> Gain1/1
  SwitchDelay/2(Turnlight_R_out) -> Gain2/1

== system ASM_Traffic_V2X_Complete_Model_2/MDLUserInterface/MotionDeskInterface/MOTION_DESK_INTERFACE/Traffic_Animation/Fellows_Animation ==
  Pos_Fellows_MainPnt_CoorSys_E[x;y;z][m] : Inport
  Angle_Fellows[x;y;z][deg] : Inport  Port=2
  Flag_FellowsUsed[0|1] : Inport  Port=3
  Bus Selector : BusSelector  OutputSignals=Pos_x_Fellows[m],Pos_y_Fellows[m],Pos_z_Fellows[m]
  Bus Selector1 : BusSelector  OutputSignals=Angle_Roll_Fellows[deg],Angle_Pitch_Fellows[deg],Angle_Yaw_Fellows[deg]
  Fellow_1 : Subsystem
  Fellow_10 : Subsystem
  Fellow_11 : Subsystem
  Fellow_12 : Subsystem
  Fellow_13 : Subsystem
  Fellow_14 : Subsystem
  Fellow_15 : Subsystem
  Fellow_2 : Subsystem
  Fellow_3 : Subsystem
  Fellow_4 : Subsystem
  Fellow_5 : Subsystem
  Fellow_6 : Subsystem
  Fellow_7 : Subsystem
  Fellow_8 : Subsystem
  Fellow_9 : Subsystem
  MDInertialCoordinateSystem : mdbs/MD_Inertial_Coordinate_System
      settings: SourceProductName=dSPACE MotionDesk Blockset
  wires:
  MDInertialCoordinateSystem/1 -> Fellow_1/1(Transform_In), Fellow_4/1(Transform_In), Fellow_5/1(Transform_In), Fellow_6/1(Transform_In), Fellow_7/1(Transform_In), Fellow_8/1(Transform_In), Fellow_9/1(Transform_In), Fellow_10/1(Transform_In), Fellow_11/1(Transform_In), Fellow_12/1(Transform_In), Fellow_13/1(Transform_In), Fellow_14/1(Transform_In), Fellow_15/1(Transform_In), Fellow_3/1(Transform_In), Fellow_2/1(Transform_In)
  Pos_Fellows_MainPnt_CoorSys_E[x;y;z][m]/1 -> Bus Selector/1
  Angle_Fellows[x;y;z][deg]/1 -> Bus Selector1/1
  Bus Selector/1 -> Fellow_4/2(Pos_x_Fellows[m]), Fellow_5/2(Pos_x_Fellows[m]), Fellow_6/2(Pos_x_Fellows[m]), Fellow_7/2(Pos_x_Fellows[m]), Fellow_8/2(Pos_x_Fellows[m]), Fellow_9/2(Pos_x_Fellows[m]), Fellow_10/2(Pos_x_Fellows[m]), Fellow_11/2(Pos_x_Fellows[m]), Fellow_12/2(Pos_x_Fellows[m]), Fellow_13/2(Pos_x_Fellows[m]), Fellow_14/2(Pos_x_Fellows[m]), Fellow_15/2(Pos_x_Fellows[m]), Fellow_3/2(Pos_x_Fellows[m]), Fellow_2/2(Pos_x_Fellows[m]), Fellow_1/2(Pos_x_Fellows[m])  "<Pos_x_Fellows[m]>"
  Bus Selector/2 -> Fellow_1/3(Pos_y_Fellows[m]), Fellow_4/3(Pos_y_Fellows[m]), Fellow_5/3(Pos_y_Fellows[m]), Fellow_6/3(Pos_y_Fellows[m]), Fellow_7/3(Pos_y_Fellows[m]), Fellow_8/3(Pos_y_Fellows[m]), Fellow_9/3(Pos_y_Fellows[m]), Fellow_10/3(Pos_y_Fellows[m]), Fellow_11/3(Pos_y_Fellows[m]), Fellow_12/3(Pos_y_Fellows[m]), Fellow_13/3(Pos_y_Fellows[m]), Fellow_14/3(Pos_y_Fellows[m]), Fellow_15/3(Pos_y_Fellows[m]), Fellow_3/3(Pos_y_Fellows[m]), Fellow_2/3(Pos_y_Fellows[m])  "<Pos_y_Fellows[m]>"
  Bus Selector/3 -> Fellow_1/4(Pos_z_Fellows[m]), Fellow_4/4(Pos_z_Fellows[m]), Fellow_5/4(Pos_z_Fellows[m]), Fellow_6/4(Pos_z_Fellows[m]), Fellow_7/4(Pos_z_Fellows[m]), Fellow_8/4(Pos_z_Fellows[m]), Fellow_9/4(Pos_z_Fellows[m]), Fellow_10/4(Pos_z_Fellows[m]), Fellow_11/4(Pos_z_Fellows[m]), Fellow_12/4(Pos_z_Fellows[m]), Fellow_13/4(Pos_z_Fellows[m]), Fellow_14/4(Pos_z_Fellows[m]), Fellow_15/4(Pos_z_Fellows[m]), Fellow_3/4(Pos_z_Fellows[m]), Fellow_2/4(Pos_z_Fellows[m])  "<Pos_z_Fellows[m]>"
  Bus Selector1/1 -> Fellow_1/5(Angle_Roll_Fellows[deg]), Fellow_4/5(Angle_Roll_Fellows[deg]), Fellow_5/5(Angle_Roll_Fellows[deg]), Fellow_6/5(Angle_Roll_Fellows[deg]), Fellow_7/5(Angle_Roll_Fellows[deg]), Fellow_8/5(Angle_Roll_Fellows[deg]), Fellow_9/5(Angle_Roll_Fellows[deg]), Fellow_10/5(Angle_Roll_Fellows[deg]), Fellow_11/5(Angle_Roll_Fellows[deg]), Fellow_12/5(Angle_Roll_Fellows[deg]), Fellow_13/5(Angle_Roll_Fellows[deg]), Fellow_14/5(Angle_Roll_Fellows[deg]), Fellow_15/5(Angle_Roll_Fellows[deg]), Fellow_3/5(Angle_Roll_Fellows[deg]), Fellow_2/5(Angle_Roll_Fellows[deg])  "<Angle_Roll_Fellows[deg]>"
  Bus Selector1/2 -> Fellow_1/6(Angle_Pitch_Fellows[deg]), Fellow_3/6(Angle_Pitch_Fellows[deg]), Fellow_4/6(Angle_Pitch_Fellows[deg]), Fellow_5/6(Angle_Pitch_Fellows[deg]), Fellow_6/6(Angle_Pitch_Fellows[deg]), Fellow_7/6(Angle_Pitch_Fellows[deg]), Fellow_8/6(Angle_Pitch_Fellows[deg]), Fellow_9/6(Angle_Pitch_Fellows[deg]), Fellow_10/6(Angle_Pitch_Fellows[deg]), Fellow_11/6(Angle_Pitch_Fellows[deg]), Fellow_12/6(Angle_Pitch_Fellows[deg]), Fellow_13/6(Angle_Pitch_Fellows[deg]), Fellow_14/6(Angle_Pitch_Fellows[deg]), Fellow_15/6(Angle_Pitch_Fellows[deg]), Fellow_2/6(Angle_Pitch_Fellows[deg])  "<Angle_Pitch_Fellows[deg]>"
  Bus Selector1/3 -> Fellow_1/7(Angle_Yaw_Fellows[deg]), Fellow_4/7(Angle_Yaw_Fellows[deg]), Fellow_5/7(Angle_Yaw_Fellows[deg]), Fellow_6/7(Angle_Yaw_Fellows[deg]), Fellow_7/7(Angle_Yaw_Fellows[deg]), Fellow_8/7(Angle_Yaw_Fellows[deg]), Fellow_9/7(Angle_Yaw_Fellows[deg]), Fellow_10/7(Angle_Yaw_Fellows[deg]), Fellow_11/7(Angle_Yaw_Fellows[deg]), Fellow_12/7(Angle_Yaw_Fellows[deg]), Fellow_13/7(Angle_Yaw_Fellows[deg]), Fellow_14/7(Angle_Yaw_Fellows[deg]), Fellow_15/7(Angle_Yaw_Fellows[deg]), Fellow_3/7(Angle_Yaw_Fellows[deg]), Fellow_2/7(Angle_Yaw_Fellows[deg])  "<Angle_Yaw_Fellows[deg]>"
  Flag_FellowsUsed[0|1]/1 -> Fellow_1/8(Flag_FellowUsed), Fellow_4/8(Flag_FellowUsed), Fellow_5/8(Flag_FellowUsed), Fellow_6/8(Flag_FellowUsed), Fellow_7/8(Flag_FellowUsed), Fellow_8/8(Flag_FellowUsed), Fellow_9/8(Flag_FellowUsed), Fellow_10/8(Flag_FellowUsed), Fellow_11/8(Flag_FellowUsed), Fellow_12/8(Flag_FellowUsed), Fellow_13/8(Flag_FellowUsed), Fellow_14/8(Flag_FellowUsed), Fellow_15/8(Flag_FellowUsed), Fellow_3/8(Flag_FellowUsed), Fellow_2/8(Flag_FellowUsed)

== system ASM_Traffic_V2X_Complete_Model_2/MDLUserInterface/MotionDeskInterface/MOTION_DESK_INTERFACE/Traffic_Animation/Sensors_Animation ==
  Transform_In : Inport
  Sensors_Signals : Inport  Port=2
  Sensor_Points : Subsystem
  Sw_Sensor_Animation[] : Constant
      settings: AttributesFormatString=1_Object3D\n2_Object2D\n3_TrafficSign\n4_LineSensor_Road_Lanes\n5_LineSensor_Road_Shape_Lines\n6_LineSensor_Road_Shape_ContObj\n7_LineSensor_Junction_Borders\n8_LineSensor_Junction_Shape_Lines\n9_LineSensor_Junction_Shape_ContObj\n10_Object3D_RadarEffects\n11_Object3D_CustomPoints
  wires:
  Transform_In/1 -> Sensor_Points/2(Transform_In)
  Sensors_Signals/1 -> Sensor_Points/3(Sensors_Signals)
  Sw_Sensor_Animation[]/1 -> Sensor_Points/1(Sw_Sensor_Animation[])

== system ASM_Traffic_V2X_Complete_Model_2/MDLUserInterface/SoftECU/MDL_DISP/SoftECU_ACC/ACC_Control_Mode[0OFF|1CC|2DC] ==
  In1 : Inport
  Out1 : Outport
  wires:
  In1/1 -> Out1/1

== system ASM_Traffic_V2X_Complete_Model_2/MDLUserInterface/SoftECU/MDL_DISP/SoftECU_ACC/ACC_State[0OFF|2Standby|3ON] ==
  In1 : Inport
  Out1 : Outport
  wires:
  In1/1 -> Out1/1

== system ASM_Traffic_V2X_Complete_Model_2/MDLUserInterface/SoftECU/MDL_DISP/SoftECU_ACC/AEB[0Off|1On] ==
  In1 : Inport
  Out1 : Outport
  wires:
  In1/1 -> Out1/1

== system ASM_Traffic_V2X_Complete_Model_2/MDLUserInterface/SoftECU/MDL_DISP/SoftECU_ACC/Collision[0Off|1On] ==
  In1 : Inport
  Out1 : Outport
  wires:
  In1/1 -> Out1/1

== system ASM_Traffic_V2X_Complete_Model_2/MDLUserInterface/SoftECU/MDL_DISP/SoftECU_ACC/Control_Mode_ACC[0Off|1CC|2DC] ==
  In1 : Inport
  Out1 : Outport
  wires:
  In1/1 -> Out1/1
